simulink model "Pricing_Harvey"  (R2022b)
settings: Solver=VariableStepAuto  StartTime=0.0  StopTime=100  RelTol=1e-3
settings Model: Creator=jaybee  LastModifiedBy=JayBee
settings ModelReferenceCC: EnableRefExpFcnMdlSchedulingChecks=on

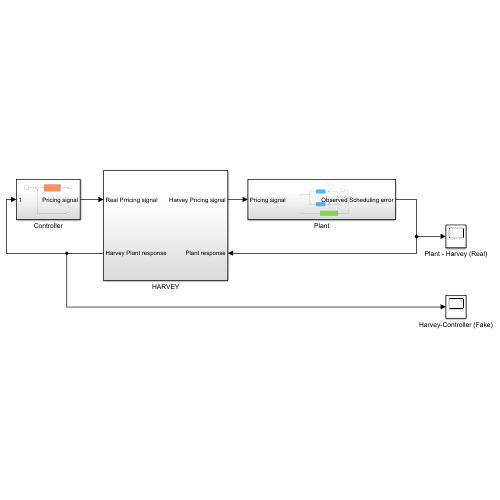
[thumbnail: Simulink's stored preview of the top-level diagram]
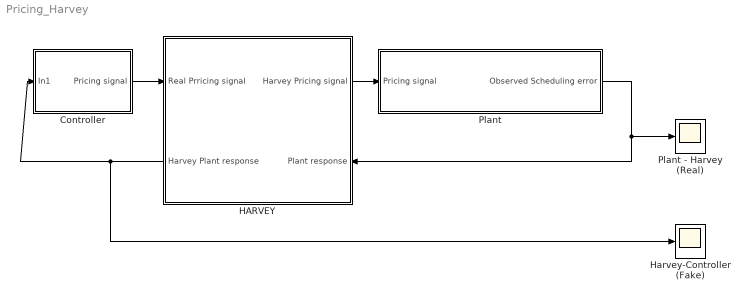
== system Pricing_Harvey ==
  Controller : Subsystem
  HARVEY : Subsystem
      settings: PortSchema="{\"entries\":[{\"content\":{\"sides\":[{\"content\":{\"connectorIds\":[\"In1\",\"Out2\"]},\"type\":\"ConnectorPlacement.EquallySpacedRectSide\",\"uuid\":\"463067e0-fab6-4de3-8785-e546c27fedfd\"},{\"content\":{\"connectorIds\":[\"Out1\",\"In2\"],\"side\":\"RIGHT\"},\"type\":\"ConnectorPlacement.EquallySpacedRectSide\",\"uuid\":\"2f3028cb-c91f-413d-a400-7bf1e9b53c29\"},{\"content\":{\"connectorIds\":[],\"side\":\"TOP\"},\"type\":\"ConnectorPlacement.EquallySpacedRectSide\",\"uuid\":\"764cf139-dacb-4138-9a8d-d633f7223dd1\"}]},\"type\":\"ConnectorPlacement.EquallySpacedConnector\",\"uuid\":\"7f787ee3-5789-43f1-8331-6a27a46020ea\"}],\"packageUris\":[\"http://schema.mathworks.com/mf0/Connector/R2020b\"],\"version\":\"1.0\"}"
  Harvey-Controller (Fake) : Scope
  Plant : Subsystem
  Plant - Harvey (Real) : Scope
  wires:
  HARVEY/2(Harvey Plant response) -> Harvey-Controller (Fake)/1, Controller/1(In1)
  Controller/1(Pricing signal) -> HARVEY/1(Real Prricing signal)
  HARVEY/1(Harvey Pricing signal) -> Plant/1(Pricing signal)
  Plant/1(Observed Scheduling error) -> Plant - Harvey (Real)/1, HARVEY/2(Plant response)

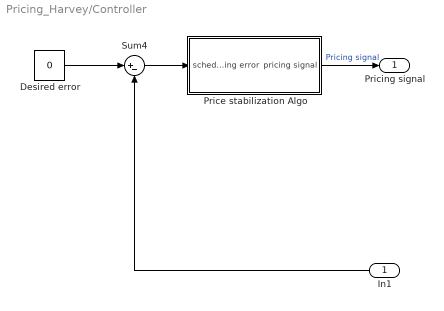
== system Pricing_Harvey/Controller ==
  In1 : Inport
  Desired error : Constant  Value=0
  Price stabilization Algo : Subsystem
  Sum4 : Sum  Inputs=|+-
  Pricing signal : Outport
  wires:
  Sum4/1 -> Price stabilization Algo/1(scheduling error)
  Desired error/1 -> Sum4/1
  Price stabilization Algo/1(pricing signal) -> Pricing signal/1  "Pricing signal"
  In1/1 -> Sum4/2

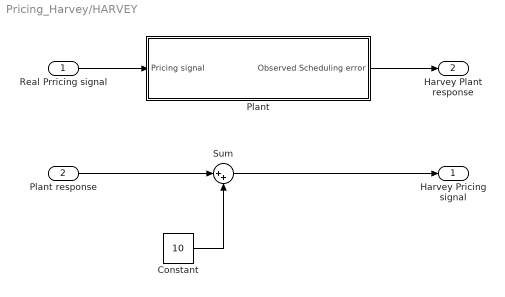
== system Pricing_Harvey/HARVEY ==
  Real Prricing signal : Inport
  Plant response : Inport  Port=2
  Constant : Constant  Value=10
  Plant : Subsystem
  Sum : Sum  Inputs=|++
  Harvey Pricing signal : Outport
  Harvey Plant response : Outport  Port=2
  wires:
  Real Prricing signal/1 -> Plant/1(Pricing signal)
  Plant/1(Observed Scheduling error) -> Harvey Plant response/1
  Plant response/1 -> Sum/1
  Sum/1 -> Harvey Pricing signal/1
  Constant/1 -> Sum/2

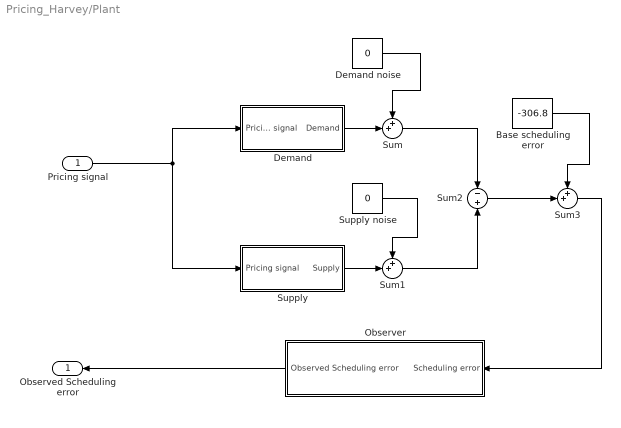
== system Pricing_Harvey/Plant ==
  Pricing signal : Inport
  Base scheduling error : Constant  Value=-306.8
  Demand : Subsystem
  Demand noise : Constant  Value=0
  Observer : Subsystem
  Sum : Sum  Inputs=++|
  Sum1 : Sum  Inputs=++|
  Sum2 : Sum  Inputs=-|+
  Sum3 : Sum  Inputs=++|
  Supply : Subsystem
  Supply noise : Constant  Value=0
  Observed Scheduling error : Outport
  wires:
  Sum1/1 -> Sum2/2
  Sum3/1 -> Observer/1(Scheduling error)
  Sum2/1 -> Sum3/2
  Supply noise/1 -> Sum1/1
  Supply/1(Supply) -> Sum1/2
  Pricing signal/1 -> Supply/1(Pricing signal), Demand/1(Pricing signal)
  Demand noise/1 -> Sum/1
  Sum/1 -> Sum2/1
  Demand/1(Demand) -> Sum/2
  Base scheduling error/1 -> Sum3/1
  Observer/1(Observed Scheduling error) -> Observed Scheduling error/1

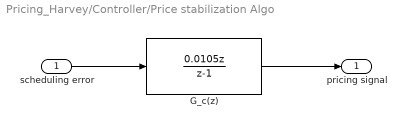
== system Pricing_Harvey/Controller/Price stabilization Algo ==
  scheduling error : Inport
  G_c(z) : DiscreteTransferFcn  Numerator=[0.0105 0]  Denominator=[1 -1]
  pricing signal : Outport
  wires:
  scheduling error/1 -> G_c(z)/1
  G_c(z)/1 -> pricing signal/1

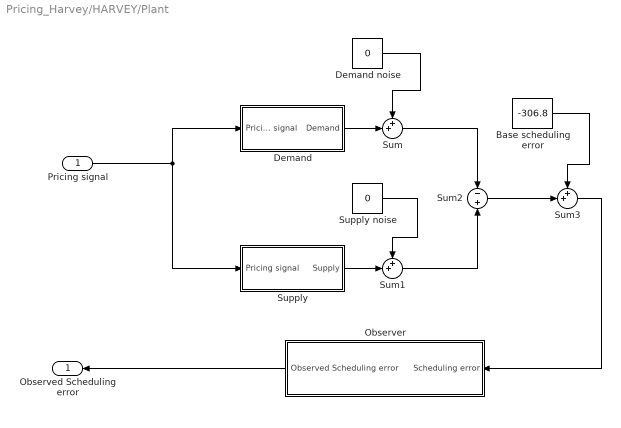
== system Pricing_Harvey/HARVEY/Plant ==
  Pricing signal : Inport
  Base scheduling error : Constant  Value=-306.8
  Demand : Subsystem
  Demand noise : Constant  Value=0
  Observer : Subsystem
  Sum : Sum  Inputs=++|
  Sum1 : Sum  Inputs=++|
  Sum2 : Sum  Inputs=-|+
  Sum3 : Sum  Inputs=++|
  Supply : Subsystem
  Supply noise : Constant  Value=0
  Observed Scheduling error : Outport
  wires:
  Sum1/1 -> Sum2/2
  Sum3/1 -> Observer/1(Scheduling error)
  Sum2/1 -> Sum3/2
  Supply noise/1 -> Sum1/1
  Supply/1(Supply) -> Sum1/2
  Pricing signal/1 -> Supply/1(Pricing signal), Demand/1(Pricing signal)
  Demand noise/1 -> Sum/1
  Sum/1 -> Sum2/1
  Demand/1(Demand) -> Sum/2
  Base scheduling error/1 -> Sum3/1
  Observer/1(Observed Scheduling error) -> Observed Scheduling error/1

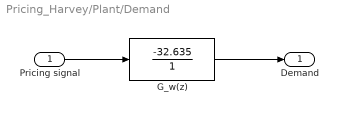
== system Pricing_Harvey/Plant/Demand ==
  Pricing signal : Inport
  G_w(z) : TransferFcn  Numerator=[-32.635]  Denominator=[0 1]
  Demand : Outport
  wires:
  Pricing signal/1 -> G_w(z)/1
  G_w(z)/1 -> Demand/1

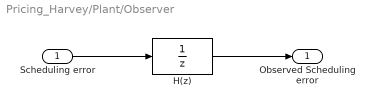
== system Pricing_Harvey/Plant/Observer ==
  Scheduling error : Inport
  H(z) : DiscreteTransferFcn  Denominator=[1 0]
  Observed Scheduling error : Outport
  wires:
  Scheduling error/1 -> H(z)/1
  H(z)/1 -> Observed Scheduling error/1

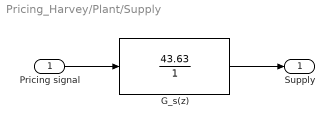
== system Pricing_Harvey/Plant/Supply ==
  Pricing signal : Inport
  G_s(z) : TransferFcn  Numerator=[43.63]  Denominator=[0 1]
  Supply : Outport
  wires:
  Pricing signal/1 -> G_s(z)/1
  G_s(z)/1 -> Supply/1

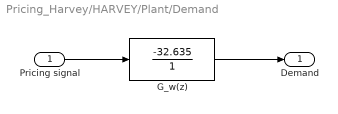
== system Pricing_Harvey/HARVEY/Plant/Demand ==
  Pricing signal : Inport
  G_w(z) : TransferFcn  Numerator=[-32.635]  Denominator=[0 1]
  Demand : Outport
  wires:
  Pricing signal/1 -> G_w(z)/1
  G_w(z)/1 -> Demand/1

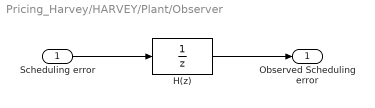
== system Pricing_Harvey/HARVEY/Plant/Observer ==
  Scheduling error : Inport
  H(z) : DiscreteTransferFcn  Denominator=[1 0]
  Observed Scheduling error : Outport
  wires:
  Scheduling error/1 -> H(z)/1
  H(z)/1 -> Observed Scheduling error/1

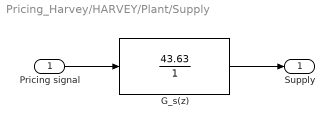
== system Pricing_Harvey/HARVEY/Plant/Supply ==
  Pricing signal : Inport
  G_s(z) : TransferFcn  Numerator=[43.63]  Denominator=[0 1]
  Supply : Outport
  wires:
  Pricing signal/1 -> G_s(z)/1
  G_s(z)/1 -> Supply/1
